simulink model "Galton_Board_v3"  (R2021a)
settings: Solver=ode23t  StartTime=0.0  StopTime=10  MaxStep=1e-3  RelTol=1e-4  AbsTol=1e-4  EnableMultiTasking=on
PreLoadFcn:
  | init_Galton_Board;
values from neighbouring files (symbols this model uses):
  D_ball = 4    [init_Galton_Board.m]
  D_peg = 4    [init_Galton_Board.m]
  H_ground = 200    [init_Galton_Board.m]
  L_peg = 12    [init_Galton_Board.m]
  X = [29.5271269861 43.8447548606 71.2892627183 40.3733262692 -83.4271156395 -32.9172730858 85.8331450424 -78.3400144776 -42.6265382176 30.9682515097 40.2739041017 95.431354449 ... (500 elements, 1x500)]    [results.mat]
undefined symbols (not defined in the file or in its folder): Y, Z
libraries: sm_lib x965, nesl_utility x3
(part 1 of 3)
settings Model: Creator=ytang  LastModifiedBy=ytang
settings SolverCC: AutoScaleAbsTol=off  AlgebraicLoopSolver=TrustRegion
settings DataIOCC: LimitDataPoints=on  MaxDataPoints=10000
settings OptimizationCC: LifeSpan=inf
settings DebuggingCC: AllowSymbolicDim=off  SFUnexpectedBacktrackingDiag=warning  SFNoUnconditionalDefaultTransitionDiag=warning  SFExecutionAtInitializationDiag=none  SFMachineParentedDataDiag=warning  ArithmeticOperatorsInVariantConditions=warning
settings SFSimCC: SimUseLocalCustomCode=off  CustomCodeUndefinedFunction=UseInterfaceOnly
settings RTWCC: RTWUseLocalCustomCode=off
settings CodeAppCC: StateflowObjectComments=on
settings GRTTargetCC: TargetLangStandard=C89/C90 (ANSI)
settings ConfigComp: CovMetricSettings=dw  CovSaveCumulativeToWorkspaceVar=on  CovSaveSingleToWorkspaceVar=on  CovExternalEMLEnable=off  CovSFcnEnable=off
settings SimscapeCC: SimscapeLogType=all  SimscapeLogSimulationStatistics=on  SimscapeLogDataHistory=10000
settings ExplorerConfigSet: InternalSimMechanicsExplorerSettings="<ExplorerConfiguration><canonicalview>default</canonicalview><AnimationSetting><BasePlaybackSpeed>1.0</BasePlaybackSpeed><PlaybackSpeedFactor>0.125</PlaybackSpeedFactor></AnimationSetting><TilePanel><TileInfo><Tiles Columns=\"1\" Count=\"1\" Rows=\"1\"><Column Weight=\"1\"/><Row Weight=\"1\"/><Tile Height=\"1\" Width=\"1\" X=\"0\" Y=\"0\"/></Tiles></TileInfo><SceneInfo><SceneViewer><BGColor><R>0.60000002384185791</R><G>0.60000002384185791</G><B>0.60000002384185791</B></BGColor><Camera><DoPerspective>off</DoPerspective><Position><X>1.84082084905140553e-09</X><Y>-0.999999967631188924</Y><Z>-0.0745000009006122621</Z></Position><Center><X>1.84082084905140553e-09</X><Y>3.23688110898112669e-08</Y><Z>-0.0745000009006122621</Z></Center><Up><X>0</X><Y>-0</Y><Z>1</Z></Up><ViewLimDist>1</ViewLimDist><YLim>0.130294995456933987</YLim><XLim>0.211521450071575828</XLim></Camera></SceneViewer></SceneInfo></TilePanel><MechEditorPanel><Cameras/><GfxPanelCameraMap/><VideoCreator><PlaybackSpeedRatio>1.0</PlaybackSpeedRatio><FrameRate>30</FrameRate><VideoFormat>Motion JPEG AVI</VideoFormat><FrameSize>auto</FrameSize></VideoCreator></MechEditorPanel></ExplorerConfiguration>"

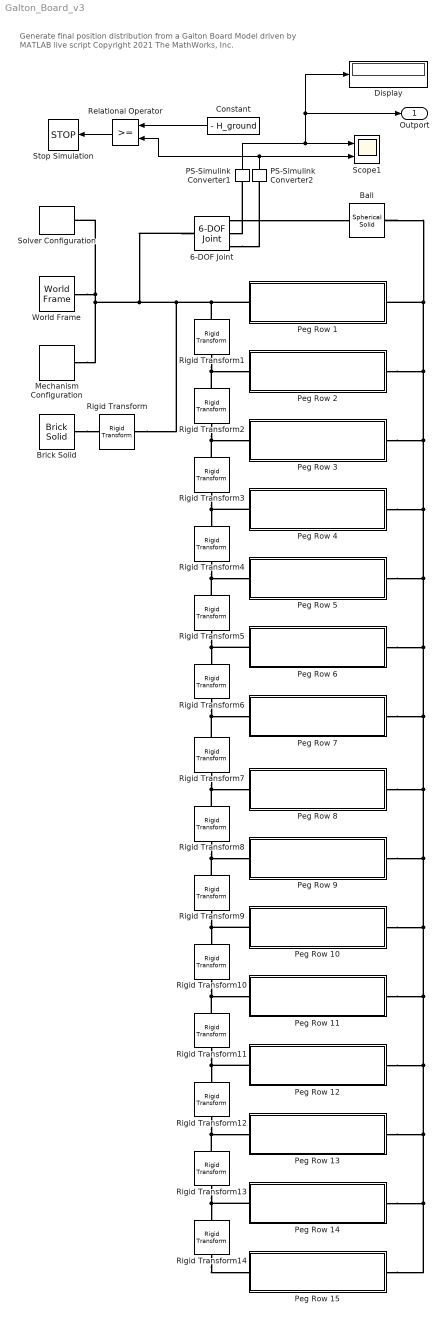
== system Galton_Board_v3 ==
  note: Generate final position distribution from a Galton Board
      |
      | Model driven by MATLAB live script
      |
      | Copyright 2021 The MathWorks, Inc.
  6-DOF Joint : sm_lib/Joints/6-DOF Joint  JointMode=Normal  SenseConstraintForce=off  SenseConstraintForceX=off  SenseConstraintForceY=off  SenseConstraintForceZ=off  SenseConstraintTorque=off  SenseConstraintTorqueX=off  SenseConstraintTorqueY=off  SenseConstraintTorqueZ=off  SenseTotalForce=off  SenseTotalForceX=off  SenseTotalForceY=off  SenseTotalForceZ=off  SenseTotalTorque=off  SenseTotalTorqueX=off  SenseTotalTorqueY=off  SenseTotalTorqueZ=off  CompositeWrenchDir=FollowerOnBase  CompositeWrenchFrame=BaseFrame  PxEquilibriumPosition=0  PxEquilibriumPositionUnits=m  PxSpringStiffness=0  PxSpringStiffnessUnits=N/m  PxDampingCoefficient=0  PxDampingCoefficientUnits=N/(m/s)  PxTorqueActuationMode=NoTorque  PxMotionActuationMode=ComputedMotion  PxSensePosition=on  PxSenseVelocity=off  PxSenseAcceleration=off  PxSenseTorqueForce=off  PxSenseLowerLimitTorqueForce=off  PxSenseUpperLimitTorqueForce=off  PxLowerLimitSpecify=off  PxLowerLimitBound=-1  PxLowerLimitBoundUnits=m  PxLowerLimitStiffness=1e6  PxLowerLimitStiffnessUnits=N/m  PxLowerLimitDamping=1e3  PxLowerLimitDampingUnits=N/(m/s)  PxLowerLimitTransitionRegionWidth=1e-4  PxLowerLimitTransitionRegionWidthUnits=m  PxUpperLimitSpecify=off  PxUpperLimitBound=1  PxUpperLimitBoundUnits=m  PxUpperLimitStiffness=1e6  PxUpperLimitStiffnessUnits=N/m  PxUpperLimitDamping=1e3  PxUpperLimitDampingUnits=N/(m/s)  PxUpperLimitTransitionRegionWidth=1e-4  PxUpperLimitTransitionRegionWidthUnits=m  PxPositionTargetSpecify=on  PxPositionTargetPriority=High  PxPositionTargetValue=x_init  PxPositionTargetValueUnits=mm  PxVelocityTargetSpecify=off  PxVelocityTargetPriority=High  PxVelocityTargetValue=0  PxVelocityTargetValueUnits=m/s  PyEquilibriumPosition=0  PyEquilibriumPositionUnits=m  PySpringStiffness=0  PySpringStiffnessUnits=N/m  PyDampingCoefficient=0  PyDampingCoefficientUnits=N/(m/s)  PyTorqueActuationMode=NoTorque  PyMotionActuationMode=ComputedMotion  PySensePosition=off  PySenseVelocity=off  PySenseAcceleration=off  PySenseTorqueForce=off  PySenseLowerLimitTorqueForce=off  PySenseUpperLimitTorqueForce=off  PyLowerLimitSpecify=off  PyLowerLimitBound=-1  PyLowerLimitBoundUnits=m  PyLowerLimitStiffness=1e6  PyLowerLimitStiffnessUnits=N/m  PyLowerLimitDamping=1e3  PyLowerLimitDampingUnits=N/(m/s)  PyLowerLimitTransitionRegionWidth=1e-4  PyLowerLimitTransitionRegionWidthUnits=m  PyUpperLimitSpecify=off  PyUpperLimitBound=1  PyUpperLimitBoundUnits=m  PyUpperLimitStiffness=1e6  PyUpperLimitStiffnessUnits=N/m  PyUpperLimitDamping=1e3  PyUpperLimitDampingUnits=N/(m/s)  PyUpperLimitTransitionRegionWidth=1e-4  PyUpperLimitTransitionRegionWidthUnits=m  PyPositionTargetSpecify=off  PyPositionTargetPriority=High  PyPositionTargetValue=0  PyPositionTargetValueUnits=m  PyVelocityTargetSpecify=off  PyVelocityTargetPriority=High  PyVelocityTargetValue=0  PyVelocityTargetValueUnits=m/s  PzEquilibriumPosition=0  PzEquilibriumPositionUnits=m  PzSpringStiffness=0  PzSpringStiffnessUnits=N/m  PzDampingCoefficient=0  PzDampingCoefficientUnits=N/(m/s)  PzTorqueActuationMode=NoTorque  PzMotionActuationMode=ComputedMotion  PzSensePosition=on  PzSenseVelocity=off  PzSenseAcceleration=off  PzSenseTorqueForce=off  PzSenseLowerLimitTorqueForce=off  PzSenseUpperLimitTorqueForce=off  PzLowerLimitSpecify=off  PzLowerLimitBound=-1  PzLowerLimitBoundUnits=m  PzLowerLimitStiffness=1e6  PzLowerLimitStiffnessUnits=N/m  PzLowerLimitDamping=1e3  PzLowerLimitDampingUnits=N/(m/s)  PzLowerLimitTransitionRegionWidth=1e-4  PzLowerLimitTransitionRegionWidthUnits=m  PzUpperLimitSpecify=off  PzUpperLimitBound=1  PzUpperLimitBoundUnits=m  PzUpperLimitStiffness=1e6  PzUpperLimitStiffnessUnits=N/m  PzUpperLimitDamping=1e3  PzUpperLimitDampingUnits=N/(m/s)  PzUpperLimitTransitionRegionWidth=1e-4  PzUpperLimitTransitionRegionWidthUnits=m  PzPositionTargetSpecify=on  PzPositionTargetPriority=High  PzPositionTargetValue=H_ball  PzPositionTargetValueUnits=mm  PzVelocityTargetSpecify=off  PzVelocityTargetPriority=High  PzVelocityTargetValue=0  PzVelocityTargetValueUnits=m/s  SphDefPosRotationMethod=None  SphDefPosRotationAngleUnits=deg  SphDefPosRotationStandardAxis=+Z  SphDefPosRotationAngle=0.0  SphDefPosRotationArbitraryAxis=[0 0 1]  SphDefPosFollAlignAxisA=+X  SphDefPosBaseAlignAxisA=+Y  SphDefPosFollAlignAxisB=+Y  SphDefPosBaseAlignAxisB=+Z  SphDefPosRotationSequenceAxes=FollowerAxes  SphDefPosRotationSequence=XYX  SphDefPosRotationSequenceAngles=[0 0 0]  SphDefPosRotationSequenceAnglesUnits=deg  SphDefPosRotationMatrix=[1 0 0; 0 1 0; 0 0 1]  SphEqPosRotationMethod=None  SphEqPosRotationAngleUnits=deg  SphEqPosRotationStandardAxis=+Z  SphEqPosRotationAngle=0.0  SphEqPosRotationArbitraryAxis=[0 0 1]  SphEqPosFollAlignAxisA=+X  SphEqPosBaseAlignAxisA=+Y  SphEqPosFollAlignAxisB=+Y  SphEqPosBaseAlignAxisB=+Z  SphEqPosRotationSequenceAxes=FollowerAxes  SphEqPosRotationSequence=XYX  SphEqPosRotationSequenceAngles=[0 0 0]  SphEqPosRotationSequenceAnglesUnits=deg  SphEqPosRotationMatrix=[1 0 0; 0 1 0; 0 0 1]  SphSpringStiffness=0  SphSpringStiffnessUnits=N*m/deg  SphDampingCoefficient=0  SphDampingCoefficientUnits=N*m/(deg/s)  SphActuateTorqueX=off  SphActuateTorqueY=off  SphActuateTorqueZ=off  SphActuateTorque=off  SphTorqueActuationMode=NoTorque  SphMotionActuationMode=ComputedMotion  SphActuationFrame=BaseFrame  SphSensePosition=off  SphSenseVelocityX=off  SphSenseVelocityY=off  SphSenseVelocityZ=off  SphSenseVelocity=off  SphSenseAccelerationX=off  SphSenseAccelerationY=off  SphSenseAccelerationZ=off  SphSenseAcceleration=off  SphSenseTorqueX=off  SphSenseTorqueY=off  SphSenseTorqueZ=off  SphSenseTorqueForce=off  SphSenseLowerLimitTorqueMag=off  SphSenseUpperLimitTorqueMag=off  SphSensingFrame=BaseFrame  SphLowerLimitSpecify=off  SphLowerLimitBound=15  SphLowerLimitBoundUnits=deg  SphLowerLimitStiffness=1e4  SphLowerLimitStiffnessUnits=N*m/deg  SphLowerLimitDamping=10  SphLowerLimitDampingUnits=N*m/(deg/s)  SphLowerLimitTransitionRegionWidth=0.1  SphLowerLimitTransitionRegionWidthUnits=deg  SphUpperLimitSpecify=off  SphUpperLimitBound=45  SphUpperLimitBoundUnits=deg  SphUpperLimitStiffness=1e4  SphUpperLimitStiffnessUnits=N*m/deg  SphUpperLimitDamping=10  SphUpperLimitDampingUnits=N*m/(deg/s)  SphUpperLimitTransitionRegionWidth=0.1  SphUpperLimitTransitionRegionWidthUnits=deg  SphPositionTargetRotationMethod=None  SphPositionTargetRotationAngleUnits=deg  SphPositionTargetRotationStandardAxis=+Z  SphPositionTargetRotationAngle=0.0  SphPositionTargetRotationArbitraryAxis=[0 0 1]  SphPositionTargetFollAlignAxisA=+X  SphPositionTargetBaseAlignAxisA=+Y  SphPositionTargetFollAlignAxisB=+Y  SphPositionTargetBaseAlignAxisB=+Z  SphPositionTargetRotationSequenceAxes=FollowerAxes  SphPositionTargetRotationSequence=XYX  SphPositionTargetRotationSequenceAngles=[0 0 0]  SphPositionTargetRotationSequenceAnglesUnits=deg  SphPositionTargetRotationMatrix=[1 0 0; 0 1 0; 0 0 1]  SphPositionTargetSpecify=off  SphPositionTargetPriority=High  SphVelocityTargetValue=[0 0 0]  SphVelocityTargetValueUnits=deg/s  SphVelocityTargetSpecify=off  SphVelocityTargetPriority=High  SphVelocityTargetInFollowerFrame=on
  Ball : sm_lib/Body Elements/Spherical Solid  GraphicAmbientColor=[0.15 0.15 0.15 1.0]  BasedOnType=Density  CenterOfMass=[0 0 0]  CenterOfMassUnits=m  GraphicDiffuseColor=[1.0 0.2 0.2]  Density=1000  DensityUnits=kg/m^3  DoExposeReferenceFrame=on  GraphicEmissiveColor=[0.0 0.0 0.0 1.0]  ExportEntireGeometry=on  SerializedExposedGeometries=<ExposedGeometries><ExposedGeometry><RawGeometryId>entire</RawGeometryId><ExposedGeometryId>G</ExposedGeometryId></ExposedGeometry></ExposedGeometries>  SerializedFrames=<Frames/>  MarkerShape=Sphere  MarkerSize=10  GraphicType=FromGeometry  InertiaType=CalculateFromGeometry  Mass=1  MassUnits=kg  MomentsOfInertia=[1 1 1]  MomentsOfInertiaUnits=kg*m^2  GraphicOpacity=1.0  ProductsOfInertia=[0 0 0]  ProductsOfInertiaUnits=kg*m^2  GraphicShininess=75  GraphicSpecularColor=[0.5 0.5 0.5 1.0]  SphereRadius=D_ball/2  SphereRadiusUnits=mm  GraphicVisPropType=SimpleVisualProperties
  Brick Solid : sm_lib/Body Elements/Brick Solid  GraphicAmbientColor=[0.15 0.15 0.15 1.0]  BasedOnType=Density  BrickDimensions=[25*L_peg 6*D_peg 2]  BrickDimensionUnits=mm  CenterOfMass=[0 0 0]  CenterOfMassUnits=m  GraphicDiffuseColor=[0.5 0.5 0.5]  Density=1000  DensityUnits=kg/m^3  DoExposeReferenceFrame=on  GraphicEmissiveColor=[0.0 0.0 0.0 1.0]  ExportEntireGeometry=off  SerializedFrames=<Frames/>  MarkerShape=Sphere  MarkerSize=10  GraphicType=FromGeometry  InertiaType=CalculateFromGeometry  Mass=1  MassUnits=kg  MomentsOfInertia=[1 1 1]  MomentsOfInertiaUnits=kg*m^2  GraphicOpacity=1.0  ProductsOfInertia=[0 0 0]  ProductsOfInertiaUnits=kg*m^2  GraphicShininess=75  GraphicSpecularColor=[0.5 0.5 0.5 1.0]  GraphicVisPropType=SimpleVisualProperties
  Constant : Constant  Value=- H_ground
  Display : Display
  Mechanism Configuration : sm_lib/Utilities/Mechanism Configuration  UniformGravity=Constant  GravityVector=[0 0 -9.80665]  GravityVectorUnits=m/s^2  GravityUnits=m/s^2  LinearizationDelta=0.001  JointModeTransitionNonlinearIterations=2
  PS-Simulink Converter1 : nesl_utility/PS-Simulink Converter  PhysicalDomain=network_engine_domain  SubClassName=ps_output  LeftPortType=input  RightPortType=output  PseudoPeriodic=off  Frequencies=[]  Unit=mm  AffineConversion=off
      settings: SourceProductBaseCode=PW,SS
  PS-Simulink Converter2 : nesl_utility/PS-Simulink Converter  PhysicalDomain=network_engine_domain  SubClassName=ps_output  LeftPortType=input  RightPortType=output  PseudoPeriodic=off  Frequencies=[]  Unit=mm  AffineConversion=off
      settings: SourceProductBaseCode=PW,SS
  Peg Row 1 : Subsystem  mask{D=D_peg, L=L_peg}
      mask prompts: D "Diameter (mm)"; L "Distance (mm)"
  Peg Row 10 : Subsystem  mask{D=D_peg, L=L_peg}
      mask prompts: D "Diameter (mm)"; L "Distance (mm)"
  Peg Row 11 : Subsystem  mask{D=D_peg, L=L_peg}
      mask prompts: D "Diameter (mm)"; L "Distance (mm)"
  Peg Row 12 : Subsystem  mask{D=D_peg, L=L_peg}
      mask prompts: D "Diameter (mm)"; L "Distance (mm)"
  Peg Row 13 : Subsystem  mask{D=D_peg, L=L_peg}
      mask prompts: D "Diameter (mm)"; L "Distance (mm)"
  Peg Row 14 : Subsystem  mask{D=D_peg, L=L_peg}
      mask prompts: D "Diameter (mm)"; L "Distance (mm)"
  Peg Row 15 : Subsystem  mask{D=D_peg, L=L_peg}
      mask prompts: D "Diameter (mm)"; L "Distance (mm)"
  Peg Row 2 : Subsystem  mask{D=D_peg, L=L_peg}
      mask prompts: D "Diameter (mm)"; L "Distance (mm)"
  Peg Row 3 : Subsystem  mask{D=D_peg, L=L_peg}
      mask prompts: D "Diameter (mm)"; L "Distance (mm)"
  Peg Row 4 : Subsystem  mask{D=D_peg, L=L_peg}
      mask prompts: D "Diameter (mm)"; L "Distance (mm)"
  Peg Row 5 : Subsystem  mask{D=D_peg, L=L_peg}
      mask prompts: D "Diameter (mm)"; L "Distance (mm)"
  Peg Row 6 : Subsystem  mask{D=D_peg, L=L_peg}
      mask prompts: D "Diameter (mm)"; L "Distance (mm)"
  Peg Row 7 : Subsystem  mask{D=D_peg, L=L_peg}
      mask prompts: D "Diameter (mm)"; L "Distance (mm)"
  Peg Row 8 : Subsystem  mask{D=D_peg, L=L_peg}
      mask prompts: D "Diameter (mm)"; L "Distance (mm)"
  Peg Row 9 : Subsystem  mask{D=D_peg, L=L_peg}
      mask prompts: D "Diameter (mm)"; L "Distance (mm)"
  Relational Operator : RelationalOperator  OutDataTypeStr=boolean  RndMeth=Simplest
  Rigid Transform : sm_lib/Frames and Transforms/Rigid Transform  TranslationMethod=StandardAxis  TranslationStandardOffset=H_ground  TranslationLengthUnit=mm  TranslationStandardAxis=-Z  TranslationCartesianOffset=[0 0 0]  TranslationROffset=0  TranslationROffsetUnits=m  TranslationZOffset=0  TranslationZOffsetUnits=m  TranslationThetaOffset=0  TranslationThetaOffsetUnits=deg  RotationMethod=None  RotationAngleUnits=deg  RotationStandardAxis=+Z  RotationAngle=0.0  RotationArbitraryAxis=[0 0 1]  FollAlignAxisA=+X  BaseAlignAxisA=+Y  FollAlignAxisB=+Y  BaseAlignAxisB=+Z  RotationSequenceAxes=FollowerAxes  RotationSequence=XYX  RotationSequenceAngles=[0 0 0]  RotationSequenceAnglesUnits=deg  RotationMatrix=[1 0 0; 0 1 0; 0 0 1]
  Rigid Transform{1,3,5,7,9,11,13} (7 alike) : sm_lib/Frames and Transforms/Rigid Transform  TranslationMethod=Cartesian  TranslationStandardOffset=H_ground  TranslationLengthUnit=mm  TranslationStandardAxis=-Z  TranslationCartesianOffset=[1/2 0 -sqrt(3)/2] * L_peg  TranslationROffset=0  TranslationROffsetUnits=m  TranslationZOffset=0  TranslationZOffsetUnits=m  TranslationThetaOffset=0  TranslationThetaOffsetUnits=deg  RotationMethod=None  RotationAngleUnits=deg  RotationStandardAxis=+Z  RotationAngle=0.0  RotationArbitraryAxis=[0 0 1]  FollAlignAxisA=+X  BaseAlignAxisA=+Y  FollAlignAxisB=+Y  BaseAlignAxisB=+Z  RotationSequenceAxes=FollowerAxes  RotationSequence=XYX  RotationSequenceAngles=[0 0 0]  RotationSequenceAnglesUnits=deg  RotationMatrix=[1 0 0; 0 1 0; 0 0 1]
  Rigid Transform{2,4,6,8,10,12,14} (7 alike) : sm_lib/Frames and Transforms/Rigid Transform  TranslationMethod=Cartesian  TranslationStandardOffset=H_ground  TranslationLengthUnit=mm  TranslationStandardAxis=-Z  TranslationCartesianOffset=[-1/2 0 -sqrt(3)/2] * L_peg  TranslationROffset=0  TranslationROffsetUnits=m  TranslationZOffset=0  TranslationZOffsetUnits=m  TranslationThetaOffset=0  TranslationThetaOffsetUnits=deg  RotationMethod=None  RotationAngleUnits=deg  RotationStandardAxis=+Z  RotationAngle=0.0  RotationArbitraryAxis=[0 0 1]  FollAlignAxisA=+X  BaseAlignAxisA=+Y  FollAlignAxisB=+Y  BaseAlignAxisB=+Z  RotationSequenceAxes=FollowerAxes  RotationSequence=XYX  RotationSequenceAngles=[0 0 0]  RotationSequenceAnglesUnits=deg  RotationMatrix=[1 0 0; 0 1 0; 0 0 1]
  Scope1 : Scope  NumInputPorts=2
  Solver Configuration : nesl_utility/Solver Configuration  PhysicalDomain=network_engine_domain  SubClassName=solver  LeftPortType=input  RightPortType=generic  Tones=[]  Harmonics=[]  SimulateNoise=off  Profile=off  UseLocalSampling=off  EnableSwitchedLinearOptims=on  FrequencyDomain=off  UseCCode=off  RelTol=0.001  AbsTol=1e-06  MinStep=1e-09  ToWorkspace=off  RevertToSquareIcSolve=off  NumHomotopyIterations=100  PhasorMode=off  PhasorModeNumHarmonics=1  DoDC=off  ResidualTolerance=1e-09  UseLocalSolver=off  LocalSolverChoice=NE_BACKWARD_EULER_ADVANCER  LocalSolverSampleTime=0.001  DoFixedCost=off  MaxNonlinIter=3  MaxModeIter=2  ComputeImpulses=off  ImpulseIterations=2  LinearAlgebra=Sparse  EquationFormulation=NE_TIME_EF  DelaysMemoryBudget=1024  AutomaticFiltering=on  FilteringTimeConstant=0.001  PartitionStorageMethod=AS_NEEDED  PartitionMemoryBudget=1024  PartitionMethod=FAST
      settings: SourceProductBaseCode=PW,SS
  Stop Simulation : Stop
  World Frame : sm_lib/Frames and Transforms/World Frame
  Outport : Outport
  wires:
  Relational Operator/1 -> Stop Simulation/1
  Constant/1 -> Relational Operator/1
  PS-Simulink Converter2/1 -> Scope1/2, Relational Operator/2
  PS-Simulink Converter1/1 -> Outport/1, Display/1, Scope1/1
  connections:
  Mechanism Configuration/RConn1 -- Rigid Transform1/LConn1 -- Peg Row 1/LConn1 -- Rigid Transform/LConn1 -- 6-DOF Joint/LConn1 -- World Frame/RConn1 -- Solver Configuration/RConn1
  6-DOF Joint/RConn1 -- Ball/RConn1
  Peg Row 14/RConn1 -- Peg Row 15/RConn1 -- Peg Row 12/RConn1 -- Peg Row 11/RConn1 -- Peg Row 10/RConn1 -- Peg Row 9/RConn1 -- Peg Row 8/RConn1 -- Peg Row 7/RConn1 -- Peg Row 6/RConn1 -- Peg Row 5/RConn1 -- Ball/LConn1 -- Peg Row 1/RConn1 -- Peg Row 2/RConn1 -- Peg Row 3/RConn1 -- Peg Row 4/RConn1 -- Peg Row 13/RConn1
  Brick Solid/RConn1 -- Rigid Transform/RConn1
  6-DOF Joint/RConn2 -- PS-Simulink Converter1/LConn1
  6-DOF Joint/RConn3 -- PS-Simulink Converter2/LConn1
  Rigid Transform1/RConn1 -- Rigid Transform2/LConn1 -- Peg Row 2/LConn1
  Rigid Transform2/RConn1 -- Rigid Transform3/LConn1 -- Peg Row 3/LConn1
  Rigid Transform4/RConn1 -- Rigid Transform5/LConn1 -- Peg Row 5/LConn1
  Rigid Transform3/RConn1 -- Peg Row 4/LConn1 -- Rigid Transform4/LConn1
  Peg Row 6/LConn1 -- Rigid Transform5/RConn1 -- Rigid Transform6/LConn1
  Rigid Transform6/RConn1 -- Rigid Transform7/LConn1 -- Peg Row 7/LConn1
  Rigid Transform8/LConn1 -- Rigid Transform7/RConn1 -- Peg Row 8/LConn1
  Rigid Transform9/LConn1 -- Rigid Transform8/RConn1 -- Peg Row 9/LConn1
  Rigid Transform10/RConn1 -- Peg Row 11/LConn1 -- Rigid Transform11/LConn1
  Peg Row 10/LConn1 -- Rigid Transform9/RConn1 -- Rigid Transform10/LConn1
  Rigid Transform11/RConn1 -- Peg Row 12/LConn1 -- Rigid Transform12/LConn1
  Rigid Transform12/RConn1 -- Rigid Transform13/LConn1 -- Peg Row 13/LConn1
  Peg Row 14/LConn1 -- Rigid Transform13/RConn1 -- Rigid Transform14/LConn1
  Rigid Transform14/RConn1 -- Peg Row 15/LConn1

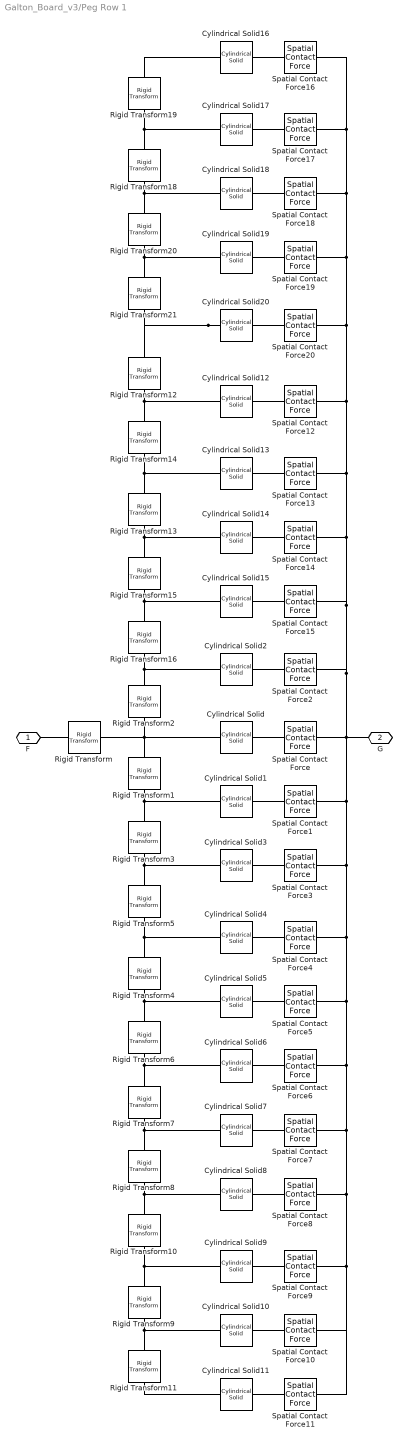
== system Galton_Board_v3/Peg Row 1 ==
  Cylindrical Solid{,1..20} (21 alike) : sm_lib/Body Elements/Cylindrical Solid  GraphicAmbientColor=[0.15 0.15 0.15 1.0]  BasedOnType=Density  CenterOfMass=[0 0 0]  CenterOfMassUnits=m  GraphicDiffuseColor=[0.5 0.5 0.5]  CylinderLength=D*4  CylinderLengthUnits=mm  CylinderRadius=D/2  CylinderRadiusUnits=mm  Density=1000  DensityUnits=kg/m^3  DoExposeReferenceFrame=on  GraphicEmissiveColor=[0.0 0.0 0.0 1.0]  ExportEntireGeometry=on  SerializedFrames=<Frames/>  MarkerShape=Sphere  MarkerSize=10  GraphicType=FromGeometry  InertiaType=CalculateFromGeometry  Mass=1  MassUnits=kg  MomentsOfInertia=[1 1 1]  MomentsOfInertiaUnits=kg*m^2  GraphicOpacity=1.0  ProductsOfInertia=[0 0 0]  ProductsOfInertiaUnits=kg*m^2  GraphicShininess=75  GraphicSpecularColor=[0.5 0.5 0.5 1.0]  GraphicVisPropType=SimpleVisualProperties
  Rigid Transform : sm_lib/Frames and Transforms/Rigid Transform  TranslationMethod=None  TranslationStandardOffset=0  TranslationLengthUnit=m  TranslationStandardAxis=+Z  TranslationCartesianOffset=[0 0 0]  TranslationROffset=0  TranslationROffsetUnits=m  TranslationZOffset=0  TranslationZOffsetUnits=m  TranslationThetaOffset=0  TranslationThetaOffsetUnits=deg  RotationMethod=StandardAxis  RotationAngleUnits=deg  RotationStandardAxis=+X  RotationAngle=90  RotationArbitraryAxis=[0 0 1]  FollAlignAxisA=+X  BaseAlignAxisA=+Y  FollAlignAxisB=+Y  BaseAlignAxisB=+Z  RotationSequenceAxes=FollowerAxes  RotationSequence=XYX  RotationSequenceAngles=[0 0 0]  RotationSequenceAnglesUnits=deg  RotationMatrix=[1 0 0; 0 1 0; 0 0 1]
  Rigid Transform{1..16,18..21} (20 alike) : sm_lib/Frames and Transforms/Rigid Transform  TranslationMethod=StandardAxis  TranslationStandardOffset=L  TranslationLengthUnit=mm  TranslationStandardAxis=+X  TranslationCartesianOffset=[0 0 0]  TranslationROffset=0  TranslationROffsetUnits=m  TranslationZOffset=0  TranslationZOffsetUnits=m  TranslationThetaOffset=0  TranslationThetaOffsetUnits=deg  RotationMethod=None  RotationAngleUnits=deg  RotationStandardAxis=+X  RotationAngle=90  RotationArbitraryAxis=[0 0 1]  FollAlignAxisA=+X  BaseAlignAxisA=+Y  FollAlignAxisB=+Y  BaseAlignAxisB=+Z  RotationSequenceAxes=FollowerAxes  RotationSequence=XYX  RotationSequenceAngles=[0 0 0]  RotationSequenceAnglesUnits=deg  RotationMatrix=[1 0 0; 0 1 0; 0 0 1]
  Spatial Contact Force{,1..20} (21 alike) : sm_lib/Forces and Torques/Spatial Contact Force  CoefficientOfDynamicFriction=0.3  CoefficientOfStaticFriction=0.5  SenseContactBaseRotation=off  SenseContactBaseTranslation=off  NormalDamping=b_scf  NormalDampingUnits=N/(m/s)  SenseContactFollowerRotation=off  SenseContactFollowerTranslation=off  SenseContactSignal=off  NormalStiffness=k_scf  NormalStiffnessUnits=N/m  FrictionalCriticalVelocity=1e-3  FrictionalCriticalVelocityUnits=m/s  ZeroCrossDetectContactStartAndEnd=off  FrictionType=SmoothStickSlip  SenseFrictionalForceMagnitude=off  SenseNormalForceMagnitude=off  NormalForceType=SmoothSpringDamper  SenseNormalVelocity=off  SenseSeparationDistance=off  SenseTangentialVelocity=off  SenseTangentialVelocityMagnitude=off  NormalTransitionRegionWidth=d_scf  NormalTransitionRegionWidthUnits=mm
  F : PMIOPort  Side=Left
  G : PMIOPort  Port=2  Side=Right
  connections:
  Rigid Transform/RConn1 -- Rigid Transform2/RConn1 -- Cylindrical Solid/RConn1 -- Rigid Transform1/LConn1
  Rigid Transform/LConn1 -- F/RConn1
  Cylindrical Solid/LConn1 -- Spatial Contact Force/LConn1
  Rigid Transform1/RConn1 -- Rigid Transform3/LConn1 -- Cylindrical Solid1/RConn1
  Spatial Contact Force19/RConn1 -- Spatial Contact Force12/RConn1 -- Spatial Contact Force13/RConn1 -- Spatial Contact Force14/RConn1 -- Spatial Contact Force4/RConn1 -- Spatial Contact Force6/RConn1 -- Spatial Contact Force7/RConn1 -- Spatial Contact Force8/RConn1 -- Spatial Contact Force9/RConn1 -- Spatial Contact Force11/RConn1 -- Spatial Contact Force10/RConn1 -- Spatial Contact Force5/RConn1 -- Spatial Contact Force3/RConn1 -- Spatial Contact Force1/RConn1 -- G/RConn1 -- Spatial Contact Force/RConn1 -- Spatial Contact Force2/RConn1 -- Spatial Contact Force15/RConn1 -- Spatial Contact Force20/RConn1 -- Spatial Contact Force18/RConn1 -- Spatial Contact Force17/RConn1 -- Spatial Contact Force16/RConn1
  Spatial Contact Force1/LConn1 -- Cylindrical Solid1/LConn1
  Spatial Contact Force2/LConn1 -- Cylindrical Solid2/LConn1
  Rigid Transform2/LConn1 -- Rigid Transform16/RConn1 -- Cylindrical Solid2/RConn1
  Spatial Contact Force3/LConn1 -- Cylindrical Solid3/LConn1
  Rigid Transform3/RConn1 -- Rigid Transform5/LConn1 -- Cylindrical Solid3/RConn1
  Rigid Transform5/RConn1 -- Rigid Transform4/LConn1 -- Cylindrical Solid4/RConn1
  Rigid Transform6/LConn1 -- Rigid Transform4/RConn1 -- Cylindrical Solid5/RConn1
  Spatial Contact Force5/LConn1 -- Cylindrical Solid5/LConn1
  Rigid Transform6/RConn1 -- Rigid Transform7/LConn1 -- Cylindrical Solid6/RConn1
  Cylindrical Solid4/LConn1 -- Spatial Contact Force4/LConn1
  Spatial Contact Force6/LConn1 -- Cylindrical Solid6/LConn1
  Rigid Transform8/LConn1 -- Rigid Transform7/RConn1 -- Cylindrical Solid7/RConn1
  Rigid Transform10/LConn1 -- Rigid Transform8/RConn1 -- Cylindrical Solid8/RConn1
  Rigid Transform9/LConn1 -- Rigid Transform10/RConn1 -- Cylindrical Solid9/RConn1
  Rigid Transform9/RConn1 -- Rigid Transform11/LConn1 -- Cylindrical Solid10/RConn1
  Spatial Contact Force11/LConn1 -- Cylindrical Solid11/LConn1
  Cylindrical Solid9/LConn1 -- Spatial Contact Force9/LConn1
  Rigid Transform11/RConn1 -- Cylindrical Solid11/RConn1
  Spatial Contact Force10/LConn1 -- Cylindrical Solid10/LConn1
  Spatial Contact Force7/LConn1 -- Cylindrical Solid7/LConn1
  Spatial Contact Force8/LConn1 -- Cylindrical Solid8/LConn1
  Rigid Transform14/LConn1 -- Rigid Transform12/RConn1 -- Cylindrical Solid12/RConn1
  Rigid Transform13/LConn1 -- Rigid Transform14/RConn1 -- Cylindrical Solid13/RConn1
  Rigid Transform13/RConn1 -- Rigid Transform15/LConn1 -- Cylindrical Solid14/RConn1
  Rigid Transform16/LConn1 -- Rigid Transform15/RConn1 -- Cylindrical Solid15/RConn1
  Spatial Contact Force15/LConn1 -- Cylindrical Solid15/LConn1
  Spatial Contact Force14/LConn1 -- Cylindrical Solid14/LConn1
  Cylindrical Solid13/LConn1 -- Spatial Contact Force13/LConn1
  Spatial Contact Force12/LConn1 -- Cylindrical Solid12/LConn1
  Rigid Transform18/RConn1 -- Rigid Transform20/LConn1 -- Cylindrical Solid18/RConn1
  Rigid Transform19/LConn1 -- Cylindrical Solid16/RConn1
  Rigid Transform18/LConn1 -- Rigid Transform19/RConn1 -- Cylindrical Solid17/RConn1
  Rigid Transform21/LConn1 -- Rigid Transform20/RConn1 -- Cylindrical Solid19/RConn1
  Cylindrical Solid20/RConn1 -- Rigid Transform12/LConn1 -- Rigid Transform21/RConn1
  Spatial Contact Force16/LConn1 -- Cylindrical Solid16/LConn1
  Cylindrical Solid17/LConn1 -- Spatial Contact Force17/LConn1
  Spatial Contact Force20/LConn1 -- Cylindrical Solid20/LConn1
  Spatial Contact Force18/LConn1 -- Cylindrical Solid18/LConn1
  Spatial Contact Force19/LConn1 -- Cylindrical Solid19/LConn1

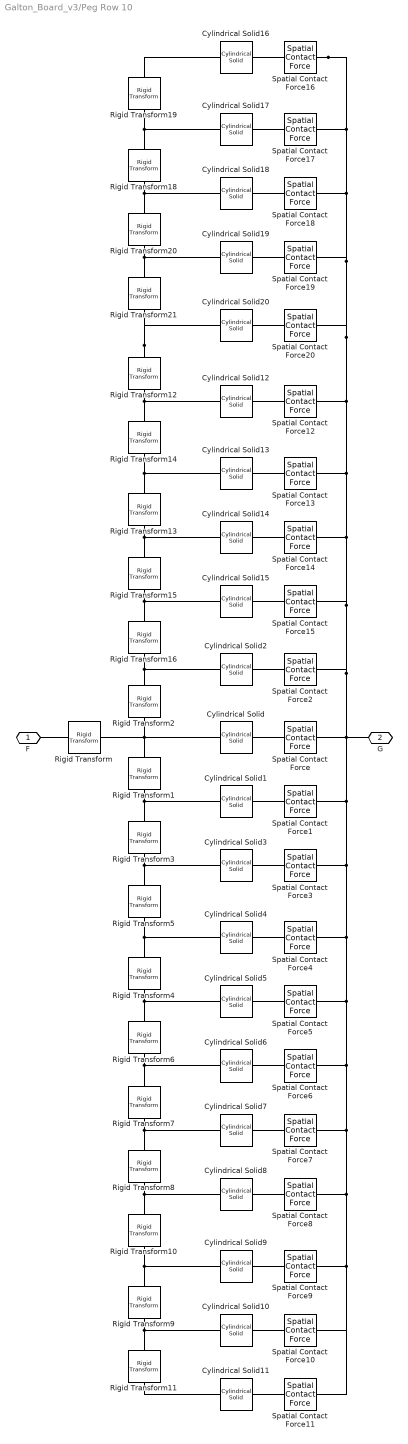
== system Galton_Board_v3/Peg Row 10 ==
  Cylindrical Solid{,1..20} (21 alike) : sm_lib/Body Elements/Cylindrical Solid  GraphicAmbientColor=[0.15 0.15 0.15 1.0]  BasedOnType=Density  CenterOfMass=[0 0 0]  CenterOfMassUnits=m  GraphicDiffuseColor=[0.5 0.5 0.5]  CylinderLength=D*4  CylinderLengthUnits=mm  CylinderRadius=D/2  CylinderRadiusUnits=mm  Density=1000  DensityUnits=kg/m^3  DoExposeReferenceFrame=on  GraphicEmissiveColor=[0.0 0.0 0.0 1.0]  ExportEntireGeometry=on  SerializedFrames=<Frames/>  MarkerShape=Sphere  MarkerSize=10  GraphicType=FromGeometry  InertiaType=CalculateFromGeometry  Mass=1  MassUnits=kg  MomentsOfInertia=[1 1 1]  MomentsOfInertiaUnits=kg*m^2  GraphicOpacity=1.0  ProductsOfInertia=[0 0 0]  ProductsOfInertiaUnits=kg*m^2  GraphicShininess=75  GraphicSpecularColor=[0.5 0.5 0.5 1.0]  GraphicVisPropType=SimpleVisualProperties
  Rigid Transform : sm_lib/Frames and Transforms/Rigid Transform  TranslationMethod=None  TranslationStandardOffset=0  TranslationLengthUnit=m  TranslationStandardAxis=+Z  TranslationCartesianOffset=[0 0 0]  TranslationROffset=0  TranslationROffsetUnits=m  TranslationZOffset=0  TranslationZOffsetUnits=m  TranslationThetaOffset=0  TranslationThetaOffsetUnits=deg  RotationMethod=StandardAxis  RotationAngleUnits=deg  RotationStandardAxis=+X  RotationAngle=90  RotationArbitraryAxis=[0 0 1]  FollAlignAxisA=+X  BaseAlignAxisA=+Y  FollAlignAxisB=+Y  BaseAlignAxisB=+Z  RotationSequenceAxes=FollowerAxes  RotationSequence=XYX  RotationSequenceAngles=[0 0 0]  RotationSequenceAnglesUnits=deg  RotationMatrix=[1 0 0; 0 1 0; 0 0 1]
  Rigid Transform{1..16,18..21} (20 alike) : sm_lib/Frames and Transforms/Rigid Transform  TranslationMethod=StandardAxis  TranslationStandardOffset=L  TranslationLengthUnit=mm  TranslationStandardAxis=+X  TranslationCartesianOffset=[0 0 0]  TranslationROffset=0  TranslationROffsetUnits=m  TranslationZOffset=0  TranslationZOffsetUnits=m  TranslationThetaOffset=0  TranslationThetaOffsetUnits=deg  RotationMethod=None  RotationAngleUnits=deg  RotationStandardAxis=+X  RotationAngle=90  RotationArbitraryAxis=[0 0 1]  FollAlignAxisA=+X  BaseAlignAxisA=+Y  FollAlignAxisB=+Y  BaseAlignAxisB=+Z  RotationSequenceAxes=FollowerAxes  RotationSequence=XYX  RotationSequenceAngles=[0 0 0]  RotationSequenceAnglesUnits=deg  RotationMatrix=[1 0 0; 0 1 0; 0 0 1]
  Spatial Contact Force{,1..20} (21 alike) : sm_lib/Forces and Torques/Spatial Contact Force  CoefficientOfDynamicFriction=0.3  CoefficientOfStaticFriction=0.5  SenseContactBaseRotation=off  SenseContactBaseTranslation=off  NormalDamping=b_scf  NormalDampingUnits=N/(m/s)  SenseContactFollowerRotation=off  SenseContactFollowerTranslation=off  SenseContactSignal=off  NormalStiffness=k_scf  NormalStiffnessUnits=N/m  FrictionalCriticalVelocity=1e-3  FrictionalCriticalVelocityUnits=m/s  ZeroCrossDetectContactStartAndEnd=off  FrictionType=SmoothStickSlip  SenseFrictionalForceMagnitude=off  SenseNormalForceMagnitude=off  NormalForceType=SmoothSpringDamper  SenseNormalVelocity=off  SenseSeparationDistance=off  SenseTangentialVelocity=off  SenseTangentialVelocityMagnitude=off  NormalTransitionRegionWidth=d_scf  NormalTransitionRegionWidthUnits=mm
  F : PMIOPort  Side=Left
  G : PMIOPort  Port=2  Side=Right
  connections:
  Spatial Contact Force19/LConn1 -- Cylindrical Solid19/LConn1
  Spatial Contact Force18/LConn1 -- Cylindrical Solid18/LConn1
  Spatial Contact Force20/LConn1 -- Cylindrical Solid20/LConn1
  Cylindrical Solid17/LConn1 -- Spatial Contact Force17/LConn1
  Spatial Contact Force16/LConn1 -- Cylindrical Solid16/LConn1
  Rigid Transform12/LConn1 -- Cylindrical Solid20/RConn1 -- Rigid Transform21/RConn1
  Rigid Transform20/RConn1 -- Rigid Transform21/LConn1 -- Cylindrical Solid19/RConn1
  Rigid Transform19/RConn1 -- Rigid Transform18/LConn1 -- Cylindrical Solid17/RConn1
  Rigid Transform19/LConn1 -- Cylindrical Solid16/RConn1
  Rigid Transform20/LConn1 -- Rigid Transform18/RConn1 -- Cylindrical Solid18/RConn1
  Spatial Contact Force12/LConn1 -- Cylindrical Solid12/LConn1
  Cylindrical Solid13/LConn1 -- Spatial Contact Force13/LConn1
  Spatial Contact Force14/LConn1 -- Cylindrical Solid14/LConn1
  Spatial Contact Force15/LConn1 -- Cylindrical Solid15/LConn1
  Rigid Transform15/RConn1 -- Rigid Transform16/LConn1 -- Cylindrical Solid15/RConn1
  Rigid Transform15/LConn1 -- Rigid Transform13/RConn1 -- Cylindrical Solid14/RConn1
  Rigid Transform14/RConn1 -- Rigid Transform13/LConn1 -- Cylindrical Solid13/RConn1
  Rigid Transform12/RConn1 -- Rigid Transform14/LConn1 -- Cylindrical Solid12/RConn1
  Spatial Contact Force8/LConn1 -- Cylindrical Solid8/LConn1
  Spatial Contact Force7/LConn1 -- Cylindrical Solid7/LConn1
  Spatial Contact Force10/LConn1 -- Cylindrical Solid10/LConn1
  Rigid Transform11/RConn1 -- Cylindrical Solid11/RConn1
  Cylindrical Solid9/LConn1 -- Spatial Contact Force9/LConn1
  Spatial Contact Force11/LConn1 -- Cylindrical Solid11/LConn1
  Rigid Transform11/LConn1 -- Rigid Transform9/RConn1 -- Cylindrical Solid10/RConn1
  Rigid Transform10/RConn1 -- Rigid Transform9/LConn1 -- Cylindrical Solid9/RConn1
  Rigid Transform8/RConn1 -- Rigid Transform10/LConn1 -- Cylindrical Solid8/RConn1
  Rigid Transform7/RConn1 -- Rigid Transform8/LConn1 -- Cylindrical Solid7/RConn1
  Spatial Contact Force6/LConn1 -- Cylindrical Solid6/LConn1
  Cylindrical Solid4/LConn1 -- Spatial Contact Force4/LConn1
  Rigid Transform7/LConn1 -- Rigid Transform6/RConn1 -- Cylindrical Solid6/RConn1
  Spatial Contact Force5/LConn1 -- Cylindrical Solid5/LConn1
  Rigid Transform4/RConn1 -- Rigid Transform6/LConn1 -- Cylindrical Solid5/RConn1
  Rigid Transform4/LConn1 -- Rigid Transform5/RConn1 -- Cylindrical Solid4/RConn1
  Rigid Transform5/LConn1 -- Rigid Transform3/RConn1 -- Cylindrical Solid3/RConn1
  Spatial Contact Force3/LConn1 -- Cylindrical Solid3/LConn1
  Rigid Transform16/RConn1 -- Cylindrical Solid2/RConn1 -- Rigid Transform2/LConn1
  Spatial Contact Force2/LConn1 -- Cylindrical Solid2/LConn1
  Spatial Contact Force1/LConn1 -- Cylindrical Solid1/LConn1
  Spatial Contact Force16/RConn1 -- Spatial Contact Force17/RConn1 -- Spatial Contact Force18/RConn1 -- Spatial Contact Force19/RConn1 -- Spatial Contact Force20/RConn1 -- Spatial Contact Force15/RConn1 -- Spatial Contact Force2/RConn1 -- Spatial Contact Force/RConn1 -- G/RConn1 -- Spatial Contact Force1/RConn1 -- Spatial Contact Force3/RConn1 -- Spatial Contact Force5/RConn1 -- Spatial Contact Force10/RConn1 -- Spatial Contact Force11/RConn1 -- Spatial Contact Force9/RConn1 -- Spatial Contact Force8/RConn1 -- Spatial Contact Force7/RConn1 -- Spatial Contact Force6/RConn1 -- Spatial Contact Force4/RConn1 -- Spatial Contact Force14/RConn1 -- Spatial Contact Force13/RConn1 -- Spatial Contact Force12/RConn1
  Rigid Transform3/LConn1 -- Rigid Transform1/RConn1 -- Cylindrical Solid1/RConn1
  Cylindrical Solid/LConn1 -- Spatial Contact Force/LConn1
  Rigid Transform/LConn1 -- F/RConn1
  Rigid Transform2/RConn1 -- Rigid Transform1/LConn1 -- Cylindrical Solid/RConn1 -- Rigid Transform/RConn1

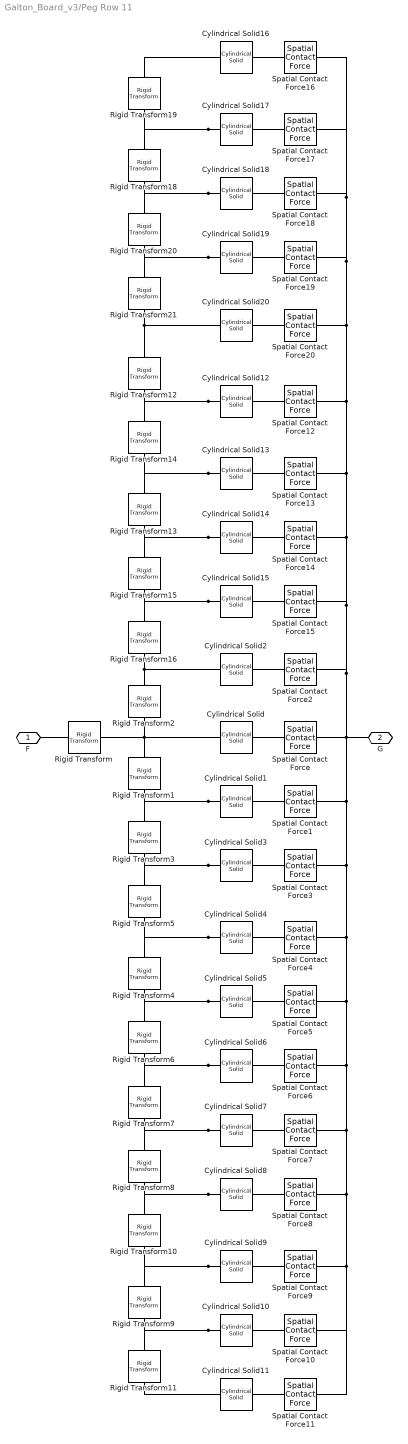
== system Galton_Board_v3/Peg Row 11 ==
  Cylindrical Solid{,1..20} (21 alike) : sm_lib/Body Elements/Cylindrical Solid  GraphicAmbientColor=[0.15 0.15 0.15 1.0]  BasedOnType=Density  CenterOfMass=[0 0 0]  CenterOfMassUnits=m  GraphicDiffuseColor=[0.5 0.5 0.5]  CylinderLength=D*4  CylinderLengthUnits=mm  CylinderRadius=D/2  CylinderRadiusUnits=mm  Density=1000  DensityUnits=kg/m^3  DoExposeReferenceFrame=on  GraphicEmissiveColor=[0.0 0.0 0.0 1.0]  ExportEntireGeometry=on  SerializedFrames=<Frames/>  MarkerShape=Sphere  MarkerSize=10  GraphicType=FromGeometry  InertiaType=CalculateFromGeometry  Mass=1  MassUnits=kg  MomentsOfInertia=[1 1 1]  MomentsOfInertiaUnits=kg*m^2  GraphicOpacity=1.0  ProductsOfInertia=[0 0 0]  ProductsOfInertiaUnits=kg*m^2  GraphicShininess=75  GraphicSpecularColor=[0.5 0.5 0.5 1.0]  GraphicVisPropType=SimpleVisualProperties
  Rigid Transform : sm_lib/Frames and Transforms/Rigid Transform  TranslationMethod=None  TranslationStandardOffset=0  TranslationLengthUnit=m  TranslationStandardAxis=+Z  TranslationCartesianOffset=[0 0 0]  TranslationROffset=0  TranslationROffsetUnits=m  TranslationZOffset=0  TranslationZOffsetUnits=m  TranslationThetaOffset=0  TranslationThetaOffsetUnits=deg  RotationMethod=StandardAxis  RotationAngleUnits=deg  RotationStandardAxis=+X  RotationAngle=90  RotationArbitraryAxis=[0 0 1]  FollAlignAxisA=+X  BaseAlignAxisA=+Y  FollAlignAxisB=+Y  BaseAlignAxisB=+Z  RotationSequenceAxes=FollowerAxes  RotationSequence=XYX  RotationSequenceAngles=[0 0 0]  RotationSequenceAnglesUnits=deg  RotationMatrix=[1 0 0; 0 1 0; 0 0 1]
  Rigid Transform{1..16,18..21} (20 alike) : sm_lib/Frames and Transforms/Rigid Transform  TranslationMethod=StandardAxis  TranslationStandardOffset=L  TranslationLengthUnit=mm  TranslationStandardAxis=+X  TranslationCartesianOffset=[0 0 0]  TranslationROffset=0  TranslationROffsetUnits=m  TranslationZOffset=0  TranslationZOffsetUnits=m  TranslationThetaOffset=0  TranslationThetaOffsetUnits=deg  RotationMethod=None  RotationAngleUnits=deg  RotationStandardAxis=+X  RotationAngle=90  RotationArbitraryAxis=[0 0 1]  FollAlignAxisA=+X  BaseAlignAxisA=+Y  FollAlignAxisB=+Y  BaseAlignAxisB=+Z  RotationSequenceAxes=FollowerAxes  RotationSequence=XYX  RotationSequenceAngles=[0 0 0]  RotationSequenceAnglesUnits=deg  RotationMatrix=[1 0 0; 0 1 0; 0 0 1]
  Spatial Contact Force{,1..20} (21 alike) : sm_lib/Forces and Torques/Spatial Contact Force  CoefficientOfDynamicFriction=0.3  CoefficientOfStaticFriction=0.5  SenseContactBaseRotation=off  SenseContactBaseTranslation=off  NormalDamping=b_scf  NormalDampingUnits=N/(m/s)  SenseContactFollowerRotation=off  SenseContactFollowerTranslation=off  SenseContactSignal=off  NormalStiffness=k_scf  NormalStiffnessUnits=N/m  FrictionalCriticalVelocity=1e-3  FrictionalCriticalVelocityUnits=m/s  ZeroCrossDetectContactStartAndEnd=off  FrictionType=SmoothStickSlip  SenseFrictionalForceMagnitude=off  SenseNormalForceMagnitude=off  NormalForceType=SmoothSpringDamper  SenseNormalVelocity=off  SenseSeparationDistance=off  SenseTangentialVelocity=off  SenseTangentialVelocityMagnitude=off  NormalTransitionRegionWidth=d_scf  NormalTransitionRegionWidthUnits=mm
  F : PMIOPort  Side=Left
  G : PMIOPort  Port=2  Side=Right
  connections:
  Rigid Transform/RConn1 -- Cylindrical Solid/RConn1 -- Rigid Transform1/LConn1 -- Rigid Transform2/RConn1
  Rigid Transform/LConn1 -- F/RConn1
  Cylindrical Solid/LConn1 -- Spatial Contact Force/LConn1
  Cylindrical Solid1/RConn1 -- Rigid Transform1/RConn1 -- Rigid Transform3/LConn1
  Spatial Contact Force12/RConn1 -- Spatial Contact Force13/RConn1 -- Spatial Contact Force14/RConn1 -- Spatial Contact Force4/RConn1 -- Spatial Contact Force6/RConn1 -- Spatial Contact Force7/RConn1 -- Spatial Contact Force8/RConn1 -- Spatial Contact Force9/RConn1 -- Spatial Contact Force11/RConn1 -- Spatial Contact Force10/RConn1 -- Spatial Contact Force5/RConn1 -- Spatial Contact Force3/RConn1 -- Spatial Contact Force1/RConn1 -- G/RConn1 -- Spatial Contact Force/RConn1 -- Spatial Contact Force2/RConn1 -- Spatial Contact Force15/RConn1 -- Spatial Contact Force20/RConn1 -- Spatial Contact Force19/RConn1 -- Spatial Contact Force18/RConn1 -- Spatial Contact Force17/RConn1 -- Spatial Contact Force16/RConn1
  Spatial Contact Force1/LConn1 -- Cylindrical Solid1/LConn1
  Spatial Contact Force2/LConn1 -- Cylindrical Solid2/LConn1
  Rigid Transform2/LConn1 -- Cylindrical Solid2/RConn1 -- Rigid Transform16/RConn1
  Spatial Contact Force3/LConn1 -- Cylindrical Solid3/LConn1
  Cylindrical Solid3/RConn1 -- Rigid Transform3/RConn1 -- Rigid Transform5/LConn1
  Cylindrical Solid4/RConn1 -- Rigid Transform5/RConn1 -- Rigid Transform4/LConn1
  Cylindrical Solid5/RConn1 -- Rigid Transform6/LConn1 -- Rigid Transform4/RConn1
  Spatial Contact Force5/LConn1 -- Cylindrical Solid5/LConn1
  Cylindrical Solid6/RConn1 -- Rigid Transform6/RConn1 -- Rigid Transform7/LConn1
  Cylindrical Solid4/LConn1 -- Spatial Contact Force4/LConn1
  Spatial Contact Force6/LConn1 -- Cylindrical Solid6/LConn1
  Cylindrical Solid7/RConn1 -- Rigid Transform8/LConn1 -- Rigid Transform7/RConn1
  Cylindrical Solid8/RConn1 -- Rigid Transform10/LConn1 -- Rigid Transform8/RConn1
  Cylindrical Solid9/RConn1 -- Rigid Transform9/LConn1 -- Rigid Transform10/RConn1
  Cylindrical Solid10/RConn1 -- Rigid Transform9/RConn1 -- Rigid Transform11/LConn1
  Spatial Contact Force11/LConn1 -- Cylindrical Solid11/LConn1
  Cylindrical Solid9/LConn1 -- Spatial Contact Force9/LConn1
  Rigid Transform11/RConn1 -- Cylindrical Solid11/RConn1
  Spatial Contact Force10/LConn1 -- Cylindrical Solid10/LConn1
  Spatial Contact Force7/LConn1 -- Cylindrical Solid7/LConn1
  Spatial Contact Force8/LConn1 -- Cylindrical Solid8/LConn1
  Cylindrical Solid12/RConn1 -- Rigid Transform14/LConn1 -- Rigid Transform12/RConn1
  Cylindrical Solid13/RConn1 -- Rigid Transform13/LConn1 -- Rigid Transform14/RConn1
  Cylindrical Solid14/RConn1 -- Rigid Transform13/RConn1 -- Rigid Transform15/LConn1
  Cylindrical Solid15/RConn1 -- Rigid Transform16/LConn1 -- Rigid Transform15/RConn1
  Spatial Contact Force15/LConn1 -- Cylindrical Solid15/LConn1
  Spatial Contact Force14/LConn1 -- Cylindrical Solid14/LConn1
  Cylindrical Solid13/LConn1 -- Spatial Contact Force13/LConn1
  Spatial Contact Force12/LConn1 -- Cylindrical Solid12/LConn1
  Cylindrical Solid18/RConn1 -- Rigid Transform18/RConn1 -- Rigid Transform20/LConn1
  Rigid Transform19/LConn1 -- Cylindrical Solid16/RConn1
  Cylindrical Solid17/RConn1 -- Rigid Transform18/LConn1 -- Rigid Transform19/RConn1
  Cylindrical Solid19/RConn1 -- Rigid Transform21/LConn1 -- Rigid Transform20/RConn1
  Rigid Transform21/RConn1 -- Cylindrical Solid20/RConn1 -- Rigid Transform12/LConn1
  Spatial Contact Force16/LConn1 -- Cylindrical Solid16/LConn1
  Cylindrical Solid17/LConn1 -- Spatial Contact Force17/LConn1
  Spatial Contact Force20/LConn1 -- Cylindrical Solid20/LConn1
  Spatial Contact Force18/LConn1 -- Cylindrical Solid18/LConn1
  Spatial Contact Force19/LConn1 -- Cylindrical Solid19/LConn1

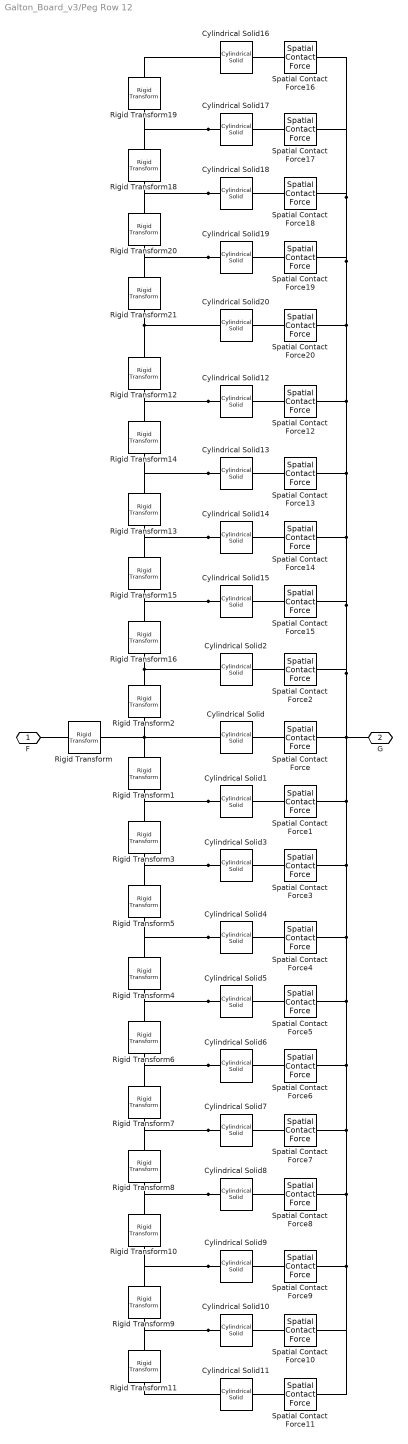
== system Galton_Board_v3/Peg Row 12 ==
  Cylindrical Solid{,1..20} (21 alike) : sm_lib/Body Elements/Cylindrical Solid  GraphicAmbientColor=[0.15 0.15 0.15 1.0]  BasedOnType=Density  CenterOfMass=[0 0 0]  CenterOfMassUnits=m  GraphicDiffuseColor=[0.5 0.5 0.5]  CylinderLength=D*4  CylinderLengthUnits=mm  CylinderRadius=D/2  CylinderRadiusUnits=mm  Density=1000  DensityUnits=kg/m^3  DoExposeReferenceFrame=on  GraphicEmissiveColor=[0.0 0.0 0.0 1.0]  ExportEntireGeometry=on  SerializedFrames=<Frames/>  MarkerShape=Sphere  MarkerSize=10  GraphicType=FromGeometry  InertiaType=CalculateFromGeometry  Mass=1  MassUnits=kg  MomentsOfInertia=[1 1 1]  MomentsOfInertiaUnits=kg*m^2  GraphicOpacity=1.0  ProductsOfInertia=[0 0 0]  ProductsOfInertiaUnits=kg*m^2  GraphicShininess=75  GraphicSpecularColor=[0.5 0.5 0.5 1.0]  GraphicVisPropType=SimpleVisualProperties
  Rigid Transform : sm_lib/Frames and Transforms/Rigid Transform  TranslationMethod=None  TranslationStandardOffset=0  TranslationLengthUnit=m  TranslationStandardAxis=+Z  TranslationCartesianOffset=[0 0 0]  TranslationROffset=0  TranslationROffsetUnits=m  TranslationZOffset=0  TranslationZOffsetUnits=m  TranslationThetaOffset=0  TranslationThetaOffsetUnits=deg  RotationMethod=StandardAxis  RotationAngleUnits=deg  RotationStandardAxis=+X  RotationAngle=90  RotationArbitraryAxis=[0 0 1]  FollAlignAxisA=+X  BaseAlignAxisA=+Y  FollAlignAxisB=+Y  BaseAlignAxisB=+Z  RotationSequenceAxes=FollowerAxes  RotationSequence=XYX  RotationSequenceAngles=[0 0 0]  RotationSequenceAnglesUnits=deg  RotationMatrix=[1 0 0; 0 1 0; 0 0 1]
  Rigid Transform{1..16,18..21} (20 alike) : sm_lib/Frames and Transforms/Rigid Transform  TranslationMethod=StandardAxis  TranslationStandardOffset=L  TranslationLengthUnit=mm  TranslationStandardAxis=+X  TranslationCartesianOffset=[0 0 0]  TranslationROffset=0  TranslationROffsetUnits=m  TranslationZOffset=0  TranslationZOffsetUnits=m  TranslationThetaOffset=0  TranslationThetaOffsetUnits=deg  RotationMethod=None  RotationAngleUnits=deg  RotationStandardAxis=+X  RotationAngle=90  RotationArbitraryAxis=[0 0 1]  FollAlignAxisA=+X  BaseAlignAxisA=+Y  FollAlignAxisB=+Y  BaseAlignAxisB=+Z  RotationSequenceAxes=FollowerAxes  RotationSequence=XYX  RotationSequenceAngles=[0 0 0]  RotationSequenceAnglesUnits=deg  RotationMatrix=[1 0 0; 0 1 0; 0 0 1]
  Spatial Contact Force{,1..20} (21 alike) : sm_lib/Forces and Torques/Spatial Contact Force  CoefficientOfDynamicFriction=0.3  CoefficientOfStaticFriction=0.5  SenseContactBaseRotation=off  SenseContactBaseTranslation=off  NormalDamping=b_scf  NormalDampingUnits=N/(m/s)  SenseContactFollowerRotation=off  SenseContactFollowerTranslation=off  SenseContactSignal=off  NormalStiffness=k_scf  NormalStiffnessUnits=N/m  FrictionalCriticalVelocity=1e-3  FrictionalCriticalVelocityUnits=m/s  ZeroCrossDetectContactStartAndEnd=off  FrictionType=SmoothStickSlip  SenseFrictionalForceMagnitude=off  SenseNormalForceMagnitude=off  NormalForceType=SmoothSpringDamper  SenseNormalVelocity=off  SenseSeparationDistance=off  SenseTangentialVelocity=off  SenseTangentialVelocityMagnitude=off  NormalTransitionRegionWidth=d_scf  NormalTransitionRegionWidthUnits=mm
  F : PMIOPort  Side=Left
  G : PMIOPort  Port=2  Side=Right
  connections:
  Rigid Transform/RConn1 -- Cylindrical Solid/RConn1 -- Rigid Transform1/LConn1 -- Rigid Transform2/RConn1
  Rigid Transform/LConn1 -- F/RConn1
  Cylindrical Solid/LConn1 -- Spatial Contact Force/LConn1
  Cylindrical Solid1/RConn1 -- Rigid Transform1/RConn1 -- Rigid Transform3/LConn1
  Spatial Contact Force12/RConn1 -- Spatial Contact Force13/RConn1 -- Spatial Contact Force14/RConn1 -- Spatial Contact Force4/RConn1 -- Spatial Contact Force6/RConn1 -- Spatial Contact Force7/RConn1 -- Spatial Contact Force8/RConn1 -- Spatial Contact Force9/RConn1 -- Spatial Contact Force11/RConn1 -- Spatial Contact Force10/RConn1 -- Spatial Contact Force5/RConn1 -- Spatial Contact Force3/RConn1 -- Spatial Contact Force1/RConn1 -- G/RConn1 -- Spatial Contact Force/RConn1 -- Spatial Contact Force2/RConn1 -- Spatial Contact Force15/RConn1 -- Spatial Contact Force20/RConn1 -- Spatial Contact Force19/RConn1 -- Spatial Contact Force18/RConn1 -- Spatial Contact Force17/RConn1 -- Spatial Contact Force16/RConn1
  Spatial Contact Force1/LConn1 -- Cylindrical Solid1/LConn1
  Spatial Contact Force2/LConn1 -- Cylindrical Solid2/LConn1
  Rigid Transform2/LConn1 -- Cylindrical Solid2/RConn1 -- Rigid Transform16/RConn1
  Spatial Contact Force3/LConn1 -- Cylindrical Solid3/LConn1
  Cylindrical Solid3/RConn1 -- Rigid Transform3/RConn1 -- Rigid Transform5/LConn1
  Cylindrical Solid4/RConn1 -- Rigid Transform5/RConn1 -- Rigid Transform4/LConn1
  Cylindrical Solid5/RConn1 -- Rigid Transform6/LConn1 -- Rigid Transform4/RConn1
  Spatial Contact Force5/LConn1 -- Cylindrical Solid5/LConn1
  Cylindrical Solid6/RConn1 -- Rigid Transform6/RConn1 -- Rigid Transform7/LConn1
  Cylindrical Solid4/LConn1 -- Spatial Contact Force4/LConn1
  Spatial Contact Force6/LConn1 -- Cylindrical Solid6/LConn1
  Cylindrical Solid7/RConn1 -- Rigid Transform8/LConn1 -- Rigid Transform7/RConn1
  Cylindrical Solid8/RConn1 -- Rigid Transform10/LConn1 -- Rigid Transform8/RConn1
  Cylindrical Solid9/RConn1 -- Rigid Transform9/LConn1 -- Rigid Transform10/RConn1
  Cylindrical Solid10/RConn1 -- Rigid Transform9/RConn1 -- Rigid Transform11/LConn1
  Spatial Contact Force11/LConn1 -- Cylindrical Solid11/LConn1
  Cylindrical Solid9/LConn1 -- Spatial Contact Force9/LConn1
  Rigid Transform11/RConn1 -- Cylindrical Solid11/RConn1
  Spatial Contact Force10/LConn1 -- Cylindrical Solid10/LConn1
  Spatial Contact Force7/LConn1 -- Cylindrical Solid7/LConn1
  Spatial Contact Force8/LConn1 -- Cylindrical Solid8/LConn1
  Cylindrical Solid12/RConn1 -- Rigid Transform14/LConn1 -- Rigid Transform12/RConn1
  Cylindrical Solid13/RConn1 -- Rigid Transform13/LConn1 -- Rigid Transform14/RConn1
  Cylindrical Solid14/RConn1 -- Rigid Transform13/RConn1 -- Rigid Transform15/LConn1
  Cylindrical Solid15/RConn1 -- Rigid Transform16/LConn1 -- Rigid Transform15/RConn1
  Spatial Contact Force15/LConn1 -- Cylindrical Solid15/LConn1
  Spatial Contact Force14/LConn1 -- Cylindrical Solid14/LConn1
  Cylindrical Solid13/LConn1 -- Spatial Contact Force13/LConn1
  Spatial Contact Force12/LConn1 -- Cylindrical Solid12/LConn1
  Cylindrical Solid18/RConn1 -- Rigid Transform18/RConn1 -- Rigid Transform20/LConn1
  Rigid Transform19/LConn1 -- Cylindrical Solid16/RConn1
  Cylindrical Solid17/RConn1 -- Rigid Transform18/LConn1 -- Rigid Transform19/RConn1
  Cylindrical Solid19/RConn1 -- Rigid Transform21/LConn1 -- Rigid Transform20/RConn1
  Rigid Transform21/RConn1 -- Cylindrical Solid20/RConn1 -- Rigid Transform12/LConn1
  Spatial Contact Force16/LConn1 -- Cylindrical Solid16/LConn1
  Cylindrical Solid17/LConn1 -- Spatial Contact Force17/LConn1
  Spatial Contact Force20/LConn1 -- Cylindrical Solid20/LConn1
  Spatial Contact Force18/LConn1 -- Cylindrical Solid18/LConn1
  Spatial Contact Force19/LConn1 -- Cylindrical Solid19/LConn1
